simulink model "VehicleSilSimulation"  (R2024a)
settings: configuration reference "standardSILConfiguraitonParams" (kept outside this file)
undefined symbols (not defined in the file or in its folder): controllerArmed, Earth, EngineCommandBus, opts, referenceLatitude_deg, referenceLongitude_deg, ServosCommandBus, WGS84
libraries: simulink x3, aerolibtransform2 x2, aerolibfltsims x1, sharedtransform x1, robotcorelib x1, uavutilslib x1
settings Model: SimulationMode=accelerator  Creator=GTAR  LastModifiedBy=jerem
settings ConfigSetRef: SourceName=standardSILConfiguraitonParams  SourceLocation=Base Workspace

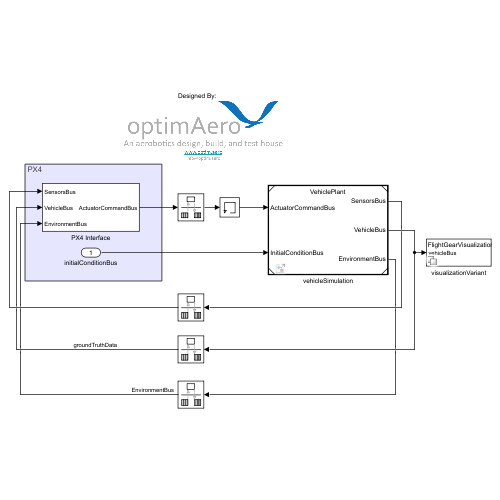
[thumbnail: Simulink's stored preview of the top-level diagram]
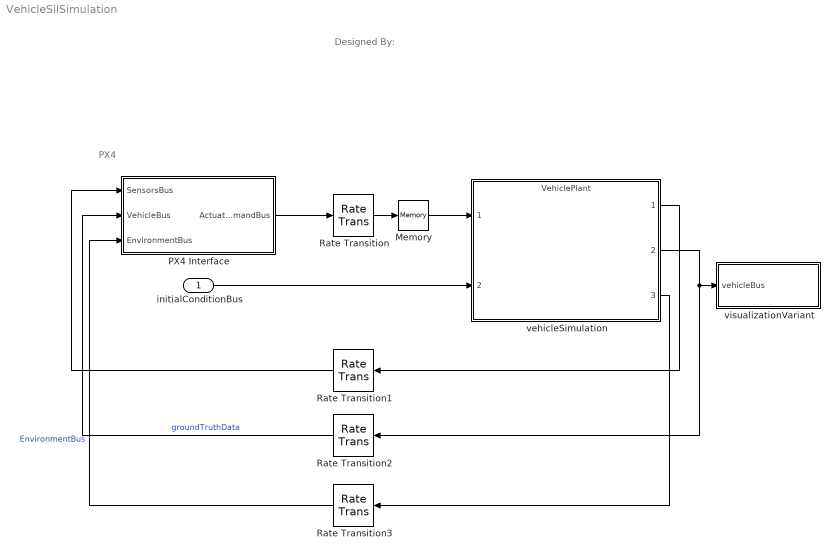
== system VehicleSilSimulation ==
  note: Designed By:
  note: PX4
  initialConditionBus : Inport
  Memory : Memory
  PX4 Interface : Subsystem  VariantControl="strcmpi(vehicleParams.type, \"F-16\") & strcmpi(vehicleParams.controllerType, \"PX4\")"
  Rate Transition{,1..3} (4 alike) : RateTransition
  vehicleSimulation : ModelReference  ModelNameDialog=VehiclePlant.slx  SimulationMode=Normal  ModelReferenceVersion=1.33
  visualizationVariant : Subsystem  Variant=on
  wires:
  initialConditionBus/1 -> vehicleSimulation/2
  vehicleSimulation/1 -> Rate Transition1/1
  vehicleSimulation/2 -> Rate Transition2/1, visualizationVariant/1(vehicleBus)
  Rate Transition/1 -> Memory/1
  Rate Transition1/1 -> PX4 Interface/1(SensorsBus)
  PX4 Interface/1(ActuatorCommandBus) -> Rate Transition/1
  Memory/1 -> vehicleSimulation/1
  Rate Transition2/1 -> PX4 Interface/2(VehicleBus)  "groundTruthData"
  vehicleSimulation/3 -> Rate Transition3/1
  Rate Transition3/1 -> PX4 Interface/3(EnvironmentBus)  "EnvironmentBus"

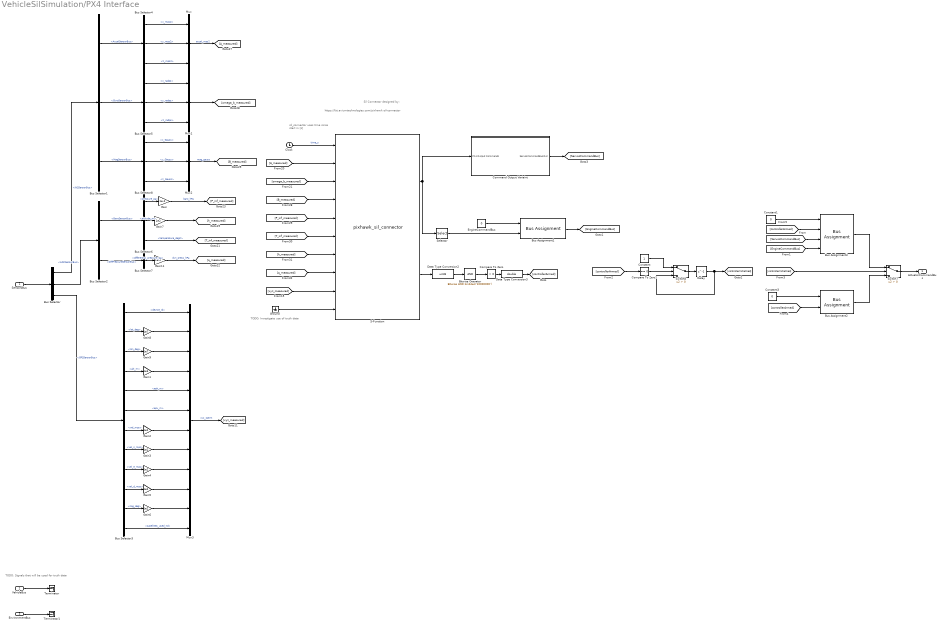
== system VehicleSilSimulation/PX4 Interface ==
  note: TODO: Signals that will be used for truth data
  note: TODO: Investigate use of truth data
  note: https://fst.aviumtechnologies.com/pixhawk-sil-connector
  note: Sil Connector designed by:
  note: sil_connector uses time since start in [s]
  SensorsBus : Inport  OutDataTypeStr=Bus: SensorsBus
  VehicleBus : Inport  Port=2  OutDataTypeStr=Bus: VehicleBus
  EnvironmentBus : Inport  Port=3  OutDataTypeStr=Bus: EnvironmentBus
  Bitwise Operator : simulink/Logic and Bit Operations/Bitwise Operator  logicop=AND  UseBitMask=on  BitMask=bin2dec('10000000')  BitMaskRealWorld=Stored Integer
  Bus Assignment1 : BusAssignment  AssignedSignals=cmdThrottle_unit
  Bus Assignment2 : BusAssignment  AssignedSignals=controllerArmed
  Bus Assignment3 : BusAssignment  AssignedSignals=controllerArmed,ServosCommandBus,EngineCommandBus
  Bus Selector : BusSelector  OutputSignals=INSSensorBus,ADCSensorBus,GPSSensorBus
  Bus Selector1 : BusSelector  OutputSignals=AccelSensorBus,GyroSensorBus,MagSensorBus
  Bus Selector2 : BusSelector  OutputSignals=BaroSensorBus,DiffPressureSensorBus
  Bus Selector3 : BusSelector  OutputSignals=device_id,lat_deg,lon_deg,alt_m,eph_m,epv_m,vel_mps,vel_n_mps,vel_e_mps,vel_d_mps,cog_deg,satellites_used_nd
  Bus Selector4 : BusSelector  OutputSignals=x_mps2,y_mps2,z_mps2
  Bus Selector5 : BusSelector  OutputSignals=x_radps,y_radps,z_radps
  Bus Selector6 : BusSelector  OutputSignals=pressure_pa,altitude_m,temperature_degC
  Bus Selector7 : BusSelector  OutputSignals=differential_pressure_pa
  Bus Selector8 : BusSelector  OutputSignals=x_Gauss,y_Gauss,z_Gauss
  Clock : Clock
  Command Output Variaint : Subsystem  Variant=on
  Compare To Zero : simulink/Logic and Bit Operations/Compare To Zero  relop=>  OutDataTypeStr=uint8
  Compare To Zero1 : simulink/Logic and Bit Operations/Compare To Zero  relop===  OutDataTypeStr=boolean
  Constant : Constant
  Constant1 : Constant  Value=0  OutDataTypeStr=Bus: ActuatorCommandBus
  Constant3 : Constant  Value=0  OutDataTypeStr=Bus: ActuatorCommandBus
  Data Type Conversion2 : DataTypeConversion  OutDataTypeStr=uint8  SaturateOnIntegerOverflow=off  RndMeth=Floor
  Data Type Conversion3 : DataTypeConversion  OutDataTypeStr=double  SaturateOnIntegerOverflow=off  RndMeth=Floor
  Delay : Delay  DelayLength=1  InitialCondition=0
  EngineCommandBus : Constant  Value=0  OutDataTypeStr=Bus: EngineCommandBus
  Gain : Gain  Gain=1e-2
  Gain1 : Gain  Gain=1e3
  Gain11 : Gain  Gain=1e-2
  Gain{2..7} (6 alike) : Gain  Gain=1e2
  Gain8 : Gain  Gain=1e7
  Gain9 : Gain  Gain=1e7
  Ground : Ground
  Mux : Mux  Inputs=3
  Mux1 : Mux  Inputs=3
  Mux2 : Mux  Inputs=3
  Mux3 : Mux  Inputs=12
  S-Function : S-Function  FunctionName=pixhawk_sil_connector  SFunctionDeploymentMode=off  EnableBusSupport=off
  Selector : Selector  InputPortWidth=16  IndexOptions=Index vector (dialog)  Indices=[1]  OutputSizes=1
  Switch7 : Switch  Criteria=u2 > Threshold  SaturateOnIntegerOverflow=off  InputSameDT=off
  Switch8 : Switch  Criteria=u2 > Threshold  SaturateOnIntegerOverflow=off  InputSameDT=off
  Terminator : Terminator
  Terminator1 : Terminator
  ActuatorCommandBus : Outport  OutDataTypeStr=Bus: ActuatorCommandBus  LockScale=on
  wires:
  Bus Selector7/1 -> Gain11/1  "<differential_pressure_pa>"
  Bus Selector4/3 -> Mux/3  "<z_mps2>"
  Bus Selector4/2 -> Mux/2  "<y_mps2>"
  Bus Selector4/1 -> Mux/1  "<x_mps2>"
  Bus Selector5/2 -> Mux1/2  "<y_radps>"
  Bus Selector6/1 -> Gain/1  "<pressure_pa>"
  Bus Selector5/1 -> Mux1/1  "<x_radps>"
  Bus Selector5/3 -> Mux1/3  "<z_radps>"
  Bus Selector3/7 -> Gain2/1  "<vel_mps>"
  Bus Selector3/5 -> Mux3/5  "<eph_m>"
  Bus Selector3/4 -> Gain1/1  "<alt_m>"
  Bus Selector3/3 -> Gain9/1  "<lon_deg>"
  Bus Selector3/2 -> Gain8/1  "<lat_deg>"
  ? -> ?
  Bus Selector2/2 -> Bus Selector7/1  "<DiffPressureSensorBus>"
  Bus Selector2/1 -> Bus Selector6/1  "<BaroSensorBus>"
  Bus Selector/2 -> Bus Selector2/1  "<ADCSensorBus>"
  Bus Selector1/2 -> Bus Selector5/1  "<GyroSensorBus>"
  Bus Selector/1 -> Bus Selector1/1  "<INSSensorBus>"
  Bus Selector/3 -> Bus Selector3/1  "<GPSSensorBus>"
  SensorsBus/1 -> Bus Selector/1
  Bus Selector1/1 -> Bus Selector4/1  "<AccelSensorBus>"
  Bus Selector1/3 -> Bus Selector8/1  "<MagSensorBus>"
  Bus Selector8/1 -> Mux2/1  "<x_Gauss>"
  Bus Selector8/2 -> Mux2/2  "<y_Gauss>"
  Bus Selector8/3 -> Mux2/3  "<z_Gauss>"
  Clock/1 -> S-Function/1  "time_s"
  Selector/1 -> Bus Assignment1/2
  S-Function/1 -> Command Output Variaint/1(PX4 Output Commands), Selector/1
  S-Function/2 -> Data Type Conversion2/1
  Data Type Conversion2/1 -> Bitwise Operator/1
  Bitwise Operator/1 -> Compare To Zero/1
  Compare To Zero/1 -> Data Type Conversion3/1
  Data Type Conversion3/1 -> [controllerArmed]
  Switch7/1 -> ActuatorCommandBus/1
  Switch8/1 -> Delay/1
  [controllerArmed] -> Compare To Zero1/1
  Constant/1 -> Switch8/1
  Compare To Zero1/1 -> Switch8/2
  Delay/1 -> Switch8/3, [controllerInitialized]
  [controllerInitialized] -> Switch7/2
  EngineCommandBus/1 -> Bus Assignment1/1
  Bus Assignment1/1 -> [EngineCommandBus]
  [controllerArmed] -> Bus Assignment2/2
  Constant3/1 -> Bus Assignment2/1
  Bus Assignment2/1 -> Switch7/3
  Constant1/1 -> Bus Assignment3/1
  [ServosCommandBus] -> Bus Assignment3/3
  [EngineCommandBus] -> Bus Assignment3/4
  [controllerArmed] -> Bus Assignment3/2
  Bus Assignment3/1 -> Switch7/1
  VehicleBus/1 -> Terminator/1
  EnvironmentBus/1 -> Terminator1/1
  [omega_b_measured] -> S-Function/3
  [B_measured] -> S-Function/4
  [P_inf_measured] -> S-Function/5
  [T_inf_measured] -> S-Function/6
  [q_measured] -> S-Function/8
  [h_measured] -> S-Function/7
  Bus Selector6/2 -> Gain7/1  "<altitude_m>"
  Bus Selector3/1 -> Mux3/1  "<device_id>"
  Gain1/1 -> Mux3/4
  Bus Selector3/6 -> Mux3/6  "<epv_m>"
  Gain2/1 -> Mux3/7
  Bus Selector3/8 -> Gain3/1  "<vel_n_mps>"
  Bus Selector3/9 -> Gain4/1  "<vel_e_mps>"
  Bus Selector3/10 -> Gain5/1  "<vel_d_mps>"
  Bus Selector3/11 -> Gain6/1  "<cog_deg>"
  Bus Selector3/12 -> Mux3/12  "<satellites_used_nd>"
  Gain3/1 -> Mux3/8
  Gain4/1 -> Mux3/9
  Gain5/1 -> Mux3/10
  Gain6/1 -> Mux3/11
  [xyz_measured] -> S-Function/9
  Mux3/1 -> [xyz_measured]  "xyz_optim"
  Gain/1 -> [P_inf_measured]  "baro_hPa"
  Gain7/1 -> [h_measured]
  Bus Selector6/3 -> [T_inf_measured]  "<temperature_degC>"
  Gain11/1 -> [q_measured]  "dyn_press_hPa"
  Mux2/1 -> [B_measured]  "mag_gauss"
  Mux1/1 -> [omega_b_measured]
  Mux/1 -> [A_measured]  "accel_mps2"
  Gain8/1 -> Mux3/2
  Gain9/1 -> Mux3/3
  [A_measured] -> S-Function/2
  Ground/1 -> S-Function/10
  Command Output Variaint/1(ServosCommandBusOut) -> [ServosCommandBus]

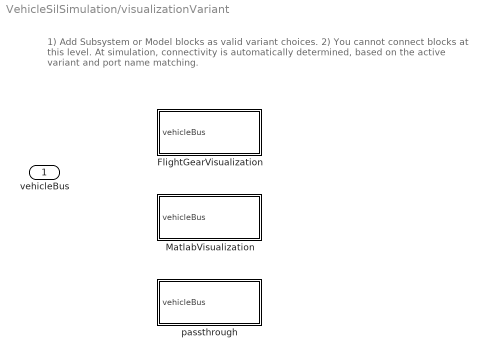
== system VehicleSilSimulation/visualizationVariant ==
  note: 1) Add Subsystem or Model blocks as valid variant choices.
      | 2) You cannot connect blocks at this level. At simulation, connectivity is automatically
      | determined, based on the active variant and port name matching.
  vehicleBus : Inport
  FlightGearVisualization : Subsystem  TreatAsAtomicUnit=on  VariantControl="strcmpi(opts.visualizationType, \"FlightGear\")"
  MatlabVisualization : Subsystem  VariantControl="strcmpi(opts.visualizationType, \"Matlab\")"
  passthrough : Subsystem  VariantControl="strcmpi(opts.visualizationType, \"PassThrough\")"

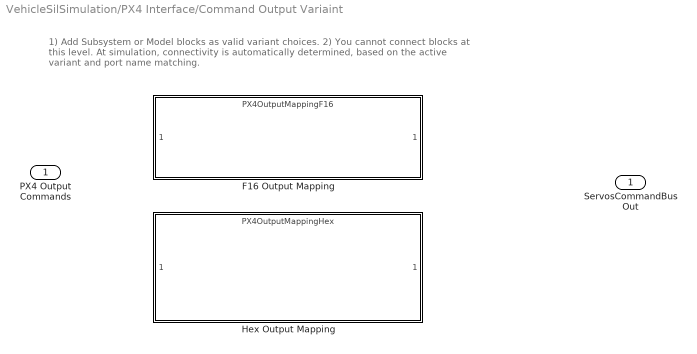
== system VehicleSilSimulation/PX4 Interface/Command Output Variaint ==
  note: 1) Add Subsystem or Model blocks as valid variant choices.
      | 2) You cannot connect blocks at this level. At simulation, connectivity is automatically
      | determined, based on the active variant and port name matching.
  PX4 Output Commands : Inport
  F16 Output Mapping : ModelReference  DisableCoverage=on  ModelNameDialog=PX4OutputMappingF16.slx  VariantControl="strcmpi(vehicleParams.type, \"F-16\") & strcmpi(vehicleParams.controllerType, \"PX4\")"  ModelReferenceVersion=1.6
  Hex Output Mapping : ModelReference  ModelNameDialog=PX4OutputMappingHex.slx  VariantControl="strcmpi(vehicleParams.type, \"hexarotor\") & strcmpi(vehicleParams.controllerType, \"PX4\")"  ModelReferenceVersion=1.5
  ServosCommandBusOut : Outport  OutDataTypeStr=Bus: ServosCommandBus

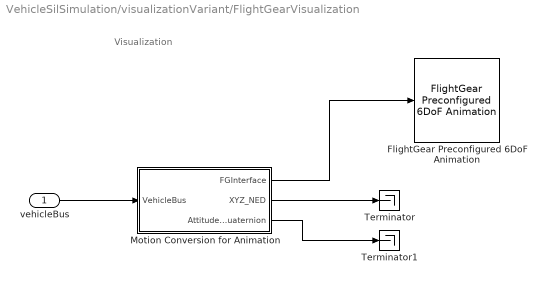
== system VehicleSilSimulation/visualizationVariant/FlightGearVisualization ==
  note: Visualization
  vehicleBus : Inport
  FlightGear Preconfigured 6DoF Animation : aerolibfltsims/FlightGear Preconfigured 6DoF Animation  xFlightGearVersion=v2019.1  DestinationIpAddress=127.0.0.1  DestinationPort=5502  SampleTime=-1  packetVersion=24
  Motion Conversion for Animation : Subsystem
      mask Display:
      | port_label('input',1,'ACBus')
      | port_label('output',1,'\lambda,L,h,\phi,\theta,\psi','texmode','on')
  Terminator : Terminator
  Terminator1 : Terminator
  wires:
  Motion Conversion for Animation/1(FGInterface) -> FlightGear Preconfigured 6DoF Animation/1
  vehicleBus/1 -> Motion Conversion for Animation/1(VehicleBus)
  Motion Conversion for Animation/2(XYZ_NED) -> Terminator/1
  Motion Conversion for Animation/3(AttitudeQuaternion) -> Terminator1/1

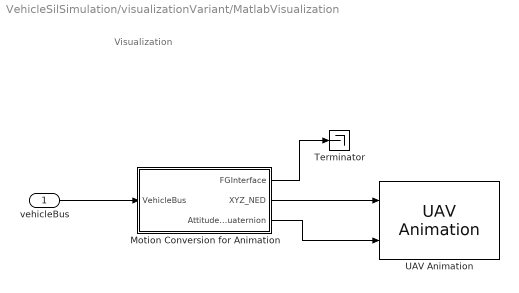
== system VehicleSilSimulation/visualizationVariant/MatlabVisualization ==
  note: Visualization
  vehicleBus : Inport
  Motion Conversion for Animation : Subsystem
      mask Display:
      | port_label('input',1,'ACBus')
      | port_label('output',1,'\lambda,L,h,\phi,\theta,\psi','texmode','on')
  Terminator : Terminator
  UAV Animation : uavutilslib/UAV Animation  UAVType=FixedWing  UAVSize=100  InertialZDirection=Down  SampleTime=-1
  wires:
  Motion Conversion for Animation/2(XYZ_NED) -> UAV Animation/1
  vehicleBus/1 -> Motion Conversion for Animation/1(VehicleBus)
  Motion Conversion for Animation/3(AttitudeQuaternion) -> UAV Animation/2
  Motion Conversion for Animation/1(FGInterface) -> Terminator/1

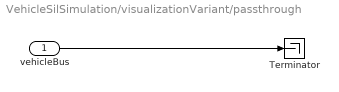
== system VehicleSilSimulation/visualizationVariant/passthrough ==
  vehicleBus : Inport
  Terminator : Terminator
  wires:
  vehicleBus/1 -> Terminator/1

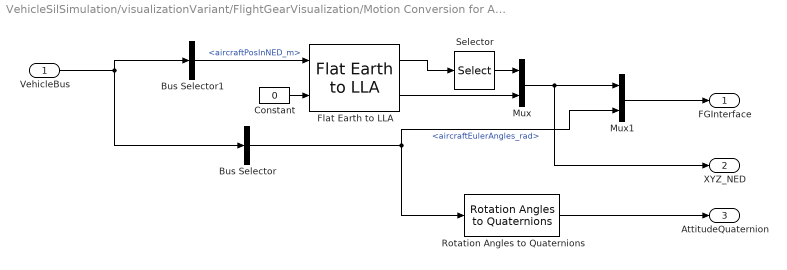
== system VehicleSilSimulation/visualizationVariant/FlightGearVisualization/Motion Conversion for Animation ==
  VehicleBus : Inport  OutDataTypeStr=Bus: VehicleBus
  Bus Selector : BusSelector  OutputSignals=BodyStates.aircraftEulerAngles_rad
  Bus Selector1 : BusSelector  OutputSignals=BodyStates.aircraftPosInNED_m
  Constant : Constant  Value=0
  Flat Earth to LLA : aerolibtransform2/Flat Earth to LLA  units=Metric (MKS)  ptype=Earth (WGS84)  F=1/298.257223563  R=6378137  refPosPort=off  LL0=[referenceLatitude_deg, referenceLongitude_deg]  psi=0
  Mux : Mux  Inputs=2
  Mux1 : Mux  Inputs=2
  Rotation Angles to Quaternions : sharedtransform/Rotation Angles to Quaternions  rotationOrder=ZYX  aMode=aMode
  Selector : Selector  IndexMode=Zero-based  InputPortWidth=2  IndexOptions=Index vector (dialog)  Indices=[1 0]  OutputSizes=1
  FGInterface : Outport  VectorParamsAs1DForOutWhenUnconnected=off
  XYZ_NED : Outport  Port=2  VectorParamsAs1DForOutWhenUnconnected=off
  AttitudeQuaternion : Outport  Port=3  VectorParamsAs1DForOutWhenUnconnected=off
  wires:
  Mux1/1 -> FGInterface/1
  Constant/1 -> Flat Earth to LLA/2
  Bus Selector/1 -> Rotation Angles to Quaternions/1, Mux1/2  "<aircraftEulerAngles_rad>"
  Flat Earth to LLA/2 -> Mux/2
  Flat Earth to LLA/1 -> Selector/1
  Bus Selector1/1 -> Flat Earth to LLA/1  "<aircraftPosInNED_m>"
  VehicleBus/1 -> Bus Selector/1, Bus Selector1/1
  Selector/1 -> Mux/1
  Mux/1 -> XYZ_NED/1, Mux1/1
  Rotation Angles to Quaternions/1 -> AttitudeQuaternion/1

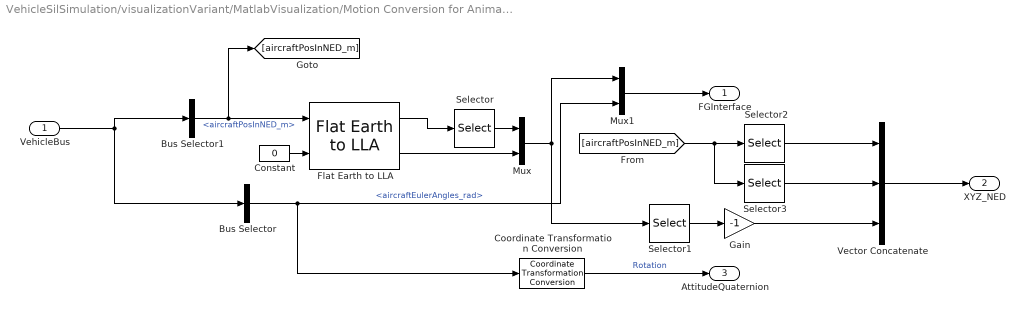
== system VehicleSilSimulation/visualizationVariant/MatlabVisualization/Motion Conversion for Animation ==
  VehicleBus : Inport  OutDataTypeStr=Bus: VehicleBus
  Bus Selector : BusSelector  OutputSignals=BodyStates.aircraftEulerAngles_rad
  Bus Selector1 : BusSelector  OutputSignals=BodyStates.aircraftPosInNED_m
  Constant : Constant  Value=0
  Coordinate Transformation Conversion : robotcorelib/Coordinate Transformation Conversion  InputRepresentation=Euler Angles  InputEulerSequence=XYZ  ShowTrVecInputPort=on  OutputRepresentation=Quaternion  OutputEulerSequence=ZYX  ShowTrVecOutputPort=on  SimulateUsing=Code generation
  Flat Earth to LLA : aerolibtransform2/Flat Earth to LLA  units=Metric (MKS)  ptype=Earth (WGS84)  F=1/298.257223563  R=6378137  refPosPort=off  LL0=[referenceLatitude_deg, referenceLongitude_deg]  psi=0
  Gain : Gain  Gain=-1
  Mux : Mux  Inputs=2
  Mux1 : Mux  Inputs=2
  Selector : Selector  IndexMode=Zero-based  InputPortWidth=2  IndexOptions=Index vector (dialog)  Indices=[1 0]  OutputSizes=1
  Selector1 : Selector  InputPortWidth=3  IndexOptions=Index vector (dialog)  Indices=3  OutputSizes=1
  Selector2 : Selector  InputPortWidth=3  IndexOptions=Index vector (dialog)  Indices=1  OutputSizes=1
  Selector3 : Selector  InputPortWidth=3  IndexOptions=Index vector (dialog)  Indices=2  OutputSizes=1
  Vector Concatenate : Concatenate  NumInputs=3
  FGInterface : Outport  VectorParamsAs1DForOutWhenUnconnected=off
  XYZ_NED : Outport  Port=2  VectorParamsAs1DForOutWhenUnconnected=off
  AttitudeQuaternion : Outport  Port=3  VectorParamsAs1DForOutWhenUnconnected=off
  wires:
  Mux1/1 -> FGInterface/1
  Constant/1 -> Flat Earth to LLA/2
  Bus Selector/1 -> Coordinate Transformation Conversion/1, Mux1/2  "<aircraftEulerAngles_rad>"
  Flat Earth to LLA/2 -> Mux/2
  Flat Earth to LLA/1 -> Selector/1
  Bus Selector1/1 -> [aircraftPosInNED_m], Flat Earth to LLA/1  "<aircraftPosInNED_m>"
  VehicleBus/1 -> Bus Selector/1, Bus Selector1/1
  Selector/1 -> Mux/1
  Mux/1 -> Selector1/1, Mux1/1
  Selector2/1 -> Vector Concatenate/1
  Selector3/1 -> Vector Concatenate/2
  Vector Concatenate/1 -> XYZ_NED/1
  Selector1/1 -> Gain/1
  Gain/1 -> Vector Concatenate/3
  [aircraftPosInNED_m] -> Selector3/1, Selector2/1
  Coordinate Transformation Conversion/1 -> AttitudeQuaternion/1  "Rotation"
